simulink model "SYS5_1"  (R2021b)
settings: Solver=ode3  StartTime=0.0  StopTime=0.5  FixedStep=1e-4  RelTol=1e-3
values from neighbouring files (symbols this model uses):
  Jn = 2*Jd    (= 0.000334)    [main.m]
  ke = (Un-R*In)/wn    (= 0.320333333333)    [main.m]
  km = Mn/In    (= 0.228971962617)    [main.m]
  ku = 20    [main.m]
  La = 10^-3 * 58    (= 0.058)    [main.m]
  R = 8.5    [main.m]
settings Model: Creator=User  LastModifiedBy=vkad
settings SolverCC: AlgebraicLoopSolver=TrustRegion
settings DebuggingCC: SFMachineParentedDataDiag=warning

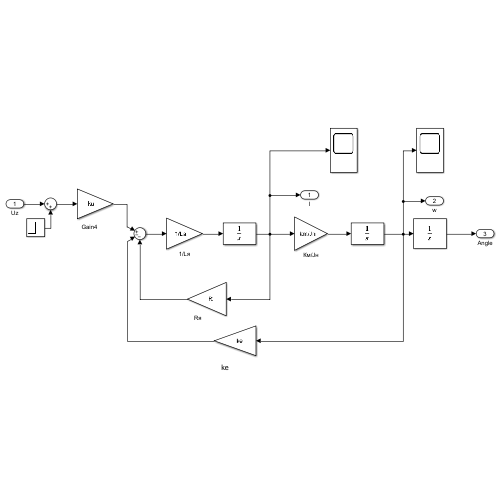
[thumbnail: Simulink's stored preview of the top-level diagram]
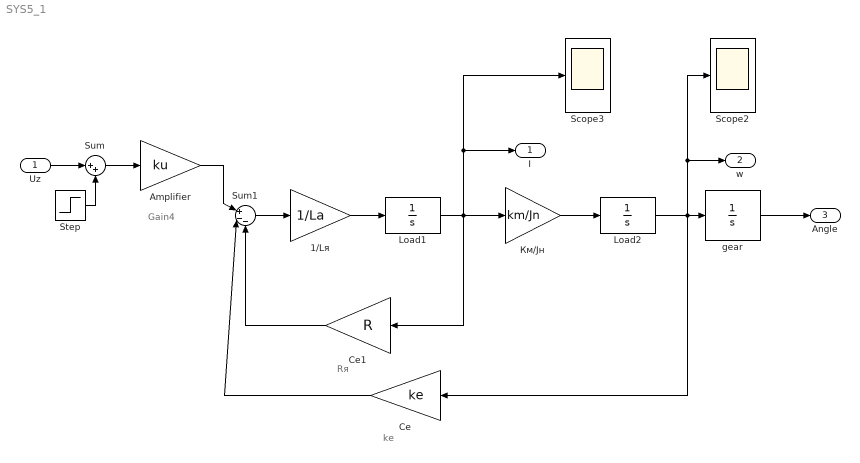
== system SYS5_1 ==
  note: kе
  note: Rя
  note: Gain4
  Uz : Inport
  1/Lя : Gain  Gain=1/La
  Amplifier : Gain  Gain=ku
  Ce : Gain  Gain=ke
  Ce1 : Gain  Gain=R
  Load1 : TransferFcn  Denominator=[1 0]
  Load2 : TransferFcn  Denominator=[1 0]
  Scope2 : Scope
  Scope3 : Scope
  Step : Step  Time=0  SampleTime=0
  Sum : Sum  Inputs=|++
  Sum1 : Sum  Inputs=|+--
  gear : TransferFcn  Numerator=1  Denominator=[1 0]
  Км/Jн : Gain  Gain=km/Jn
  I : Outport
  w : Outport  Port=2
  Angle : Outport  Port=3
  wires:
  Amplifier/1 -> Sum1/1
  Ce/1 -> Sum1/2
  Load2/1 -> Ce/1, w/1, Scope2/1, gear/1
  Sum1/1 -> 1/Lя/1
  Sum/1 -> Amplifier/1
  gear/1 -> Angle/1
  Uz/1 -> Sum/1
  1/Lя/1 -> Load1/1
  Ce1/1 -> Sum1/3
  Load1/1 -> I/1, Scope3/1, Км/Jн/1, Ce1/1
  Step/1 -> Sum/2
  Км/Jн/1 -> Load2/1
